simulink model "ClosedLoop_Test_systune"  (R2023b)
settings: Solver=VariableStepAuto  StartTime=0.0  StopTime=10.0  RelTol=1e-3
libraries: cstblocks x7
settings Model: Creator=PierluigiMeneses  LastModifiedBy=PierluigiMeneses

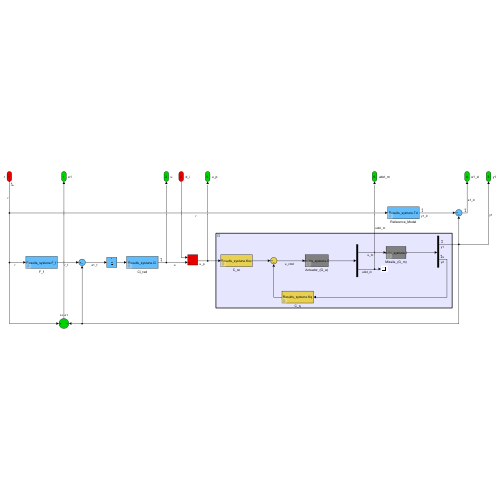
[thumbnail: Simulink's stored preview of the top-level diagram]
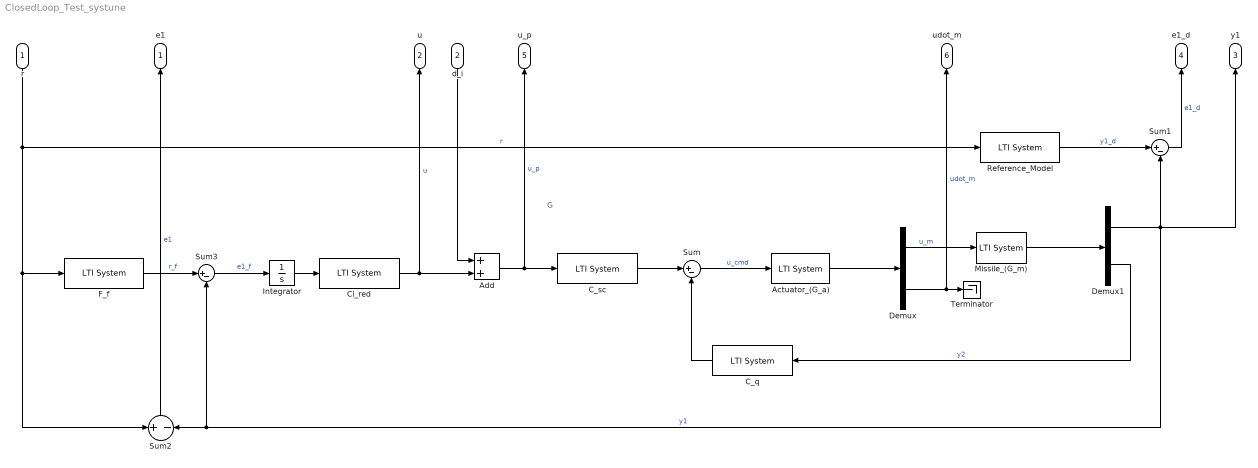
== system ClosedLoop_Test_systune ==
  note: G
  r : Inport
  d_i : Inport  Port=2
  Actuator_(G_a) : cstblocks/LTI System  sys=Results_systune.Ga  IC=[]  PadeOrder=0
  Add : Sum
  C_q : cstblocks/LTI System  sys=Results_systune.Kq  IC=[]  PadeOrder=0
  C_sc : cstblocks/LTI System  sys=Results_systune.Ksc  IC=[]  PadeOrder=0
  Ci_red : cstblocks/LTI System  sys=Results_systune.Ci  IC=[]  PadeOrder=0
  Demux : Demux  Outputs=2
  Demux1 : Demux  Outputs=2
  F_f : cstblocks/LTI System  sys=Results_systune.F_f  IC=[]  PadeOrder=0
  Integrator : Integrator
  Missile_(G_m) : cstblocks/LTI System  sys=Results_systune.Gm  IC=[]  PadeOrder=0
  Reference_Model : cstblocks/LTI System  sys=Results_systune.Td  IC=[]  PadeOrder=0
  Sum : Sum  Inputs=|+-
  Sum1 : Sum  Inputs=|+-
  Sum2 : Sum  Inputs=+|-
  Sum3 : Sum  Inputs=|+-
  Terminator : Terminator
  e1 : Outport
  u : Outport  Port=2
  y1 : Outport  Port=3
  e1_d : Outport  Port=4
  u_p : Outport  Port=5
  udot_m : Outport  Port=6
  wires:
  Sum2/1 -> e1/1  "e1"
  d_i/1 -> Add/1
  r/1 -> Reference_Model/1, Sum2/1, F_f/1  "r"
  Reference_Model/1 -> Sum1/1  "y1_d"
  Integrator/1 -> Ci_red/1
  Ci_red/1 -> Add/2, u/1  "u"
  Demux/2 -> udot_m/1, Terminator/1  "udot_m"
  Sum3/1 -> Integrator/1  "e1_f"
  Sum1/1 -> e1_d/1  "e1_d"
  Actuator_(G_a)/1 -> Demux/1
  Demux1/2 -> C_q/1  "y2"
  Sum/1 -> Actuator_(G_a)/1  "u_cmd"
  C_sc/1 -> Sum/1
  F_f/1 -> Sum3/1  "r_f"
  Demux1/1 -> y1/1, Sum1/2, Sum2/2, Sum3/2  "y1"
  Missile_(G_m)/1 -> Demux1/1
  Add/1 -> C_sc/1, u_p/1  "u_p"
  Demux/1 -> Missile_(G_m)/1  "u_m"
  C_q/1 -> Sum/2
